simulink model "gray16QAM"  (R2023a)
settings: Solver=FixedStepDiscrete  StartTime=0.0  StopTime=inf  RelTol=1e-3  AbsTol=1e-6
PreLoadFcn:
  | EbNo=3;maxNumErrs=100;maxNumBits=1e8;M=8;Tsym=.2;
libraries: simulink x2, commsink2 x2, commdigbbndam3 x2, commchan3 x1, commrandsrc3 x1
CloseFcn:
  | clear graySER grayBER graySigsOut EbNo maxNumErrs maxNumBits M Tsym
Description:
  | Gray Coded 8-PSK
  | 
  | This model shows a communications link using Gray-coded 8-PSK modulation.
settings Model: RequirementInfo=9  ExtModeTrigMode=oneshot  Creator=The MathWorks, Inc.  LastModifiedBy=athmajanvivekananthan
settings SolverCC: AutoScaleAbsTol=off  AlgebraicLoopSolver=TrustRegion
settings DataIOCC: SaveFormat=Array  SaveOutput=off  SaveTime=off  ReturnWorkspaceOutputs=off  SignalLoggingName=graySigsOut
settings OptimizationCC: BlockReduction=off  BooleanDataType=off  ReuseModelBlockBuffer=off  ExpressionDepthLimit=2147483647  InitFltsAndDblsToZero=on  EfficientMapNaN2IntZero=off  LifeSpan=inf  BufferReusableBoundary=off
settings DebuggingCC: SaveWithParameterizedLinksMsg=none  CheckExecutionContextPreStartOutputMsg=on  SignalResolutionControl=TryResolveAllWithWarning  MultiTaskDSMMsg=warning  MultiTaskCondExecSysMsg=none  SigSpecEnsureSampleTimeMsg=none  IntegerOverflowMsg=none  UnconnectedInputMsg=warning  UnconnectedOutputMsg=warning  UnconnectedLineMsg=warning  BusObjectLabelMismatch=none  StateNameClashWarn=warning  SFUnexpectedBacktrackingDiag=warning  SFNoUnconditionalDefaultTransitionDiag=warning  SFExecutionAtInitializationDiag=none  IntegerSaturationMsg=none  ArithmeticOperatorsInVariantConditions=warning
settings HardwareCC: ProdBitPerPointer=32  ProdBitPerSizeT=32  ProdBitPerPtrDiffT=32  ProdLargestAtomicFloat=None  ProdIntDivRoundTo=Undefined  ProdEndianess=Unspecified  ProdWordSize=32  ProdHWDeviceType=Specified
settings ModelReferenceCC: UpdateModelReferenceTargets=IfOutOfDate  EnableRefExpFcnMdlSchedulingChecks=on  PropagateSignalLabelsOutOfModel=off
settings SFSimCC: SimUseLocalCustomCode=off  CustomCodeUndefinedFunction=UseInterfaceOnly
settings RTWCC: RTWUseLocalCustomCode=off  DLArmComputeVersion=19.05
settings CodeAppCC: MangleLength=5  StateflowObjectComments=on
settings GRTTargetCC: TargetFcnLib=ansi_tfl_tmw.mat  TargetLangStandard=C89/C90 (ANSI)  CombineOutputUpdateFcns=off  GRTInterface=on
settings ConfigComp: CovMetricSettings=d  CovSaveCumulativeToWorkspaceVar=on  CovSaveSingleToWorkspaceVar=on  CovExternalEMLEnable=off

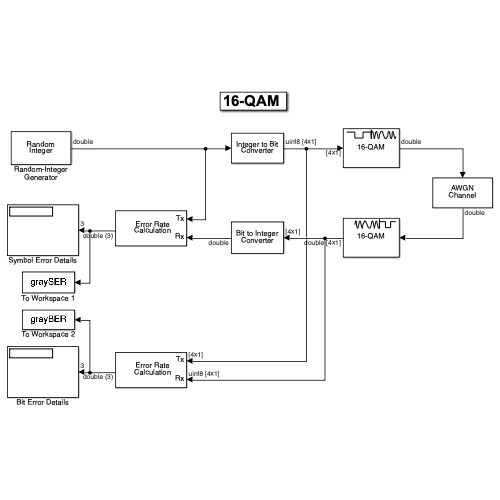
[thumbnail: Simulink's stored preview of the top-level diagram]
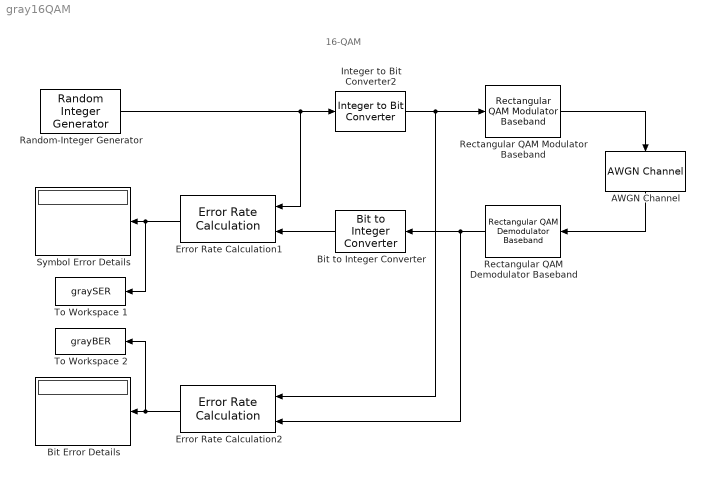
== system gray16QAM ==
  note: 16-QAM
  AWGN Channel : commchan3/AWGN Channel  LegacyMode=off  NoiseMethod="Signal to noise ratio  (Eb/No)"  noiseMode="Signal to noise ratio  (SNR)"  EbNo=EbNo  EsNo=10  SNR=10  BitsPerSymbol=log2(M)  SignalPower=1  SamplesPerSymbol=1  SymbolPeriod=1  VarianceSource=Parameter  Variance=1  RandomStream=mt19937ar with seed  Seed=67  SimulateUsing=Code generation
  Bit Error Details : Display
  Bit to Integer Converter : simulink/Logic and Bit Operations/Bit to Integer Converter  nbits=log2(M)  bitOrder=MSB first  signedOutputValues=Unsigned  outDtype=double  outDtypeSigned=Inherit via internal rule
      settings: LibrarySourceBlock=|
      | commutil2/Bit to Integer
      | Converter
  Error Rate Calculation1 : commsink2/Error Rate Calculation  N=0  st_delay=0  cp_mode=Entire frame  subframe=[]  PMode=Port  WsName=SymErrorVec  RsMode2=off  stop=off  numErr=100  maxBits=1e6
  Error Rate Calculation2 : commsink2/Error Rate Calculation  N=0  st_delay=0  cp_mode=Entire frame  subframe=[]  PMode=Port  WsName=BitErrorVec  RsMode2=off  stop=on  numErr=maxNumErrs  maxBits=maxNumBits
  Integer to Bit Converter2 : simulink/Logic and Bit Operations/Integer to Bit Converter  nbits=log2(M)  signedInputValues=Unsigned  bitOrder=MSB first  outDtype=Smallest unsigned integer
      settings: LibrarySourceBlock=|
      | commutil2/Integer to Bit
      | Converter
  Random-Integer Generator : commrandsrc3/Random Integer Generator  SetSize=8  SeedSource=Auto  Seed=0  SampleTime=1  SamplesPerFrame=1  OutputDataType=double  SimulateUsing=Interpreted execution
  Rectangular QAM Demodulator Baseband : commdigbbndam3/Rectangular QAM Demodulator Baseband  M=16  OutType=Bit  DecType=Hard decision  VarSource=Dialog  Variance=1  Dec=Gray  Mapping=[0:15]  PowType=Min. distance between symbols  MinDist=2  AvgPow=1  PeakPow=1  Ph=0  outDtype1=Smallest unsigned integer  outDtype2=Inherit via internal rule  derotateFactorWordLen=16  derotateFactorDataTypeStr=Inherit: Same word length as input  derotateFactorLastDataTypeStr=Inherit: Same word length as input  denormFactorWordLen=16  denormFactorDataTypeStr=Inherit: Same word length as input  denormFactorLastDataTypeStr=Inherit: Same word length as input  prodOutWordLen=32  prodOutOverflowMode=Wrap  prodOutRoundingMode=Floor  prodOutOvFlMode=off  prodOutOvFlModeLastStrValue=off  sumWordLen=32
  Rectangular QAM Modulator Baseband : commdigbbndam3/Rectangular QAM Modulator Baseband  M=16  InType=Bit  Enc=Gray  Mapping=[0:15]  PowType=Min. distance between symbols  MinDist=2  AvgPow=1  PeakPow=1  Ph=0  outDtype=Inherit via back propagation  outWordLen=16  outUDDataType=sfix(16)  outFracLenMode=Best precision  outFracLen=15  outDataTypeStr=Inherit: Inherit via back propagation  outLastDataTypeStr=Inherit: Inherit via back propagation
  Symbol Error Details : Display
  To Workspace 1 : ToWorkspace  VariableName=graySER  SampleTime=-1
      settings: MaxDataPoints=1
  To Workspace 2 : ToWorkspace  VariableName=grayBER  SampleTime=-1
      settings: MaxDataPoints=1
  wires:
  Error Rate Calculation2/1 -> Bit Error Details/1, To Workspace 2/1
  Error Rate Calculation1/1 -> Symbol Error Details/1, To Workspace 1/1
  Rectangular QAM Demodulator Baseband/1 -> Bit to Integer Converter/1, Error Rate Calculation2/2
  AWGN Channel/1 -> Rectangular QAM Demodulator Baseband/1
  Rectangular QAM Modulator Baseband/1 -> AWGN Channel/1
  Integer to Bit Converter2/1 -> Rectangular QAM Modulator Baseband/1, Error Rate Calculation2/1
  Bit to Integer Converter/1 -> Error Rate Calculation1/2
  Random-Integer Generator/1 -> Integer to Bit Converter2/1, Error Rate Calculation1/1
